simulink model "px42LoopCtrQGCGPS202203131707"  (R2022a)
settings: Solver=FixedStepDiscrete  StartTime=0.0  StopTime=inf  FixedStep=0.005  RelTol=1e-3  EnableMultiTasking=on
InitFcn:
  | I_x = 0.00478;
  | I_y = 0.00502;
  | I_z = 0.00736;
  | m=1;
  | L=0.11667;
undefined symbols (not defined in the file): alt, cog_rad, dev, DiscIntNeverNeededParam, eph, epv, fix_type, lat, lon, m_to_mm, Main, ms_to_cms, pwm_output0, ref_height, ref_lat, ref_lon, SampleTime, satellites_used, time_utc_usec, vel_d_m_s, vel_e_m_s, vel_m_s, vel_n_m_s, vx, vy, vz, x, y, z
libraries: simulink x26, px4uORBlib x5, sensorgpslib x1, px4lib x1, slpidlib x1, sharedtransform x1, px4Sensorslib x1
(part 3 of 3)

== system px42LoopCtrQGCGPS202203131707/Attitude controller/Subsystem1/Subsystem1/Subsystem ==
  Add1 : Sum
  Data Store Read : DataStoreRead  DataStoreName=t  IndexOptions=Index vector (dialog)  Indices=1  OutputSizes=1
  Fcn : Fcn  Expr=u(1)/(u(2)-u(3))
  Mux1 : Mux  Inputs=3
  Scope : Scope
  Switch : Switch  Threshold=5  SaturateOnIntegerOverflow=off  InputSameDT=off
  T : Constant  Value=5
  ch : Constant  Value=3
  r : Constant
  t : Constant  Value=0
  H : Outport
  wires:
  r/1 -> Add1/1
  Data Store Read/1 -> Switch/2, Mux1/3
  Mux1/1 -> Fcn/1
  ch/1 -> Mux1/1
  t/1 -> Switch/1
  T/1 -> Mux1/2
  Add1/1 -> H/1
  Fcn/1 -> Switch/3
  Switch/1 -> Scope/1, Add1/2

== system px42LoopCtrQGCGPS202203131707/Attitude controller/Subsystem6/Subsystem1/Subsystem ==
  Abs : Abs  SaturateOnIntegerOverflow=off
  Add : Sum  Inputs=+-
  Add1 : Sum
  Compare To Constant1 : simulink/Logic and Bit Operations/Compare To Constant  relop=>=  const=pi/36  OutDataTypeStr=boolean
  Data Store Memory : DataStoreMemory  DataStoreName=start_time_roll  ReadBeforeWriteMsg=warning  WriteAfterWriteMsg=warning  WriteAfterReadMsg=warning  ShowAdditionalParam=off
  Data Store Read : DataStoreRead  DataStoreName=t  IndexOptions=Index vector (dialog)  Indices=1  OutputSizes=1
  Data Store Read1 : DataStoreRead  DataStoreName=e_pitch_roll  IndexOptions=Index vector (dialog)  Indices=1  OutputSizes=1
  Data Store Read3 : DataStoreRead  DataStoreName=start_time_roll  IndexOptions=Index vector (dialog)  Indices=1  OutputSizes=1
  Data Store Read4 : DataStoreRead  DataStoreName=start_time_roll  IndexOptions=Index vector (dialog)  Indices=1  OutputSizes=1
  Display : Display
  Fcn : Fcn  Expr=u(1)/(u(2)-u(3))
  MATLAB Function : MATLAB Function  TreatAsAtomicUnit=on
  Mux1 : Mux  Inputs=3
  Scope : Scope
  T : Constant  Value=5
  ch : Constant  Value=2
  r : Constant  Value=6.001388888888889
  start_time : Subsystem
  t : Constant  Value=0
  H : Outport
  wires:
  MATLAB Function/1(y) -> Scope/1, Add1/2
  Compare To Constant1/1 -> MATLAB Function/1(e)
  Fcn/1 -> MATLAB Function/4(y1)
  t/1 -> MATLAB Function/5(y2)
  Data Store Read4/1 -> Display/1
  Data Store Read3/1 -> Add/2, MATLAB Function/3(s_t)
  Mux1/1 -> Fcn/1
  Add/1 -> Mux1/3
  ch/1 -> Mux1/1
  Data Store Read/1 -> Add/1, MATLAB Function/2(t)
  T/1 -> Mux1/2
  Abs/1 -> Compare To Constant1/1
  Data Store Read1/1 -> Abs/1
  Add1/1 -> H/1
  r/1 -> Add1/1

== system px42LoopCtrQGCGPS202203131707/Attitude controller/Subsystem7/Subsystem1/Subsystem ==
  Abs : Abs  SaturateOnIntegerOverflow=off
  Add : Sum  Inputs=+-
  Add1 : Sum
  Compare To Constant1 : simulink/Logic and Bit Operations/Compare To Constant  relop=>=  const=pi/36  OutDataTypeStr=boolean
  Data Store Memory : DataStoreMemory  DataStoreName=start_time_yaw  ReadBeforeWriteMsg=warning  WriteAfterWriteMsg=warning  WriteAfterReadMsg=warning  ShowAdditionalParam=off
  Data Store Read : DataStoreRead  DataStoreName=t  IndexOptions=Index vector (dialog)  Indices=1  OutputSizes=1
  Data Store Read1 : DataStoreRead  DataStoreName=e_pitch_yaw  IndexOptions=Index vector (dialog)  Indices=1  OutputSizes=1
  Data Store Read3 : DataStoreRead  DataStoreName=start_time_yaw  IndexOptions=Index vector (dialog)  Indices=1  OutputSizes=1
  Data Store Read4 : DataStoreRead  DataStoreName=start_time_yaw  IndexOptions=Index vector (dialog)  Indices=1  OutputSizes=1
  Display : Display
  Fcn : Fcn  Expr=u(1)/(u(2)-u(3))
  MATLAB Function : MATLAB Function  TreatAsAtomicUnit=on
  Mux1 : Mux  Inputs=3
  Scope : Scope
  T : Constant  Value=5
  ch : Constant  Value=2
  r : Constant  Value=8.00109649122807
  start_time : Subsystem
  t : Constant  Value=0
  H : Outport
  wires:
  MATLAB Function/1(y) -> Scope/1, Add1/2
  Compare To Constant1/1 -> MATLAB Function/1(e)
  Fcn/1 -> MATLAB Function/4(y1)
  t/1 -> MATLAB Function/5(y2)
  Data Store Read4/1 -> Display/1
  Data Store Read3/1 -> Add/2, MATLAB Function/3(s_t)
  Mux1/1 -> Fcn/1
  Add/1 -> Mux1/3
  ch/1 -> Mux1/1
  Data Store Read/1 -> Add/1, MATLAB Function/2(t)
  T/1 -> Mux1/2
  Abs/1 -> Compare To Constant1/1
  Data Store Read1/1 -> Abs/1
  Add1/1 -> H/1
  r/1 -> Add1/1

== system px42LoopCtrQGCGPS202203131707/Attitude controller/Subsystem/Subsystem1/Subsystem/start_time ==
  Abs1 : Abs  SaturateOnIntegerOverflow=off
  Abs2 : Abs  Commented=on  SaturateOnIntegerOverflow=off
  Add : Sum  Inputs=+-
  Add2 : Sum  Commented=on  Inputs=+-
  Compare To Constant1 : simulink/Logic and Bit Operations/Compare To Constant  relop=>=  const=4.6  OutDataTypeStr=boolean
  Compare To Constant2 : simulink/Logic and Bit Operations/Compare To Constant  relop=>=  const=pi/36  OutDataTypeStr=boolean
  Compare To Constant4 : simulink/Logic and Bit Operations/Compare To Constant  Commented=on  relop=>=  const=pi/36  OutDataTypeStr=boolean
  Compare To Constant5 : simulink/Logic and Bit Operations/Compare To Constant  Commented=on  relop=>=  const=5  OutDataTypeStr=boolean
  Data Store Read : DataStoreRead  DataStoreName=t  IndexOptions=Index vector (dialog)  Indices=1  OutputSizes=1
  Data Store Read2 : DataStoreRead  DataStoreName=e_pitch  IndexOptions=Index vector (dialog)  Indices=1  OutputSizes=1
  Data Store Read3 : DataStoreRead  DataStoreName=start_time  IndexOptions=Index vector (dialog)  Indices=1  OutputSizes=1
  Data Store Read5 : DataStoreRead  Commented=on  DataStoreName=e_pitch  IndexOptions=Index vector (dialog)  Indices=1  OutputSizes=1
  Data Store Read6 : DataStoreRead  Commented=on  DataStoreName=t  IndexOptions=Index vector (dialog)  Indices=1  OutputSizes=1
  Data Store Read7 : DataStoreRead  Commented=on  DataStoreName=start_time  IndexOptions=Index vector (dialog)  Indices=1  OutputSizes=1
  Logical Operator : Logic  AllPortsSameDT=off  OutDataTypeStr=boolean
  Logical Operator1 : Logic  Commented=on  AllPortsSameDT=off  OutDataTypeStr=boolean
  Subsystem : Subsystem
  Subsystem1 : Subsystem  Commented=on
  wires:
  Data Store Read7/1 -> Add2/2
  Abs1/1 -> Compare To Constant2/1
  Data Store Read2/1 -> Abs1/1
  Logical Operator1/1 -> Subsystem1/Trigger
  Compare To Constant5/1 -> Logical Operator1/2
  Add2/1 -> Compare To Constant5/1
  Compare To Constant4/1 -> Logical Operator1/1
  Data Store Read5/1 -> Abs2/1
  Data Store Read6/1 -> Add2/1
  Abs2/1 -> Compare To Constant4/1
  Data Store Read3/1 -> Add/2
  Data Store Read/1 -> Add/1
  Add/1 -> Compare To Constant1/1
  Compare To Constant2/1 -> Logical Operator/1
  Compare To Constant1/1 -> Logical Operator/2
  Logical Operator/1 -> Subsystem/Trigger

== system px42LoopCtrQGCGPS202203131707/Attitude controller/Subsystem6/Subsystem1/Subsystem/start_time ==
  Abs1 : Abs  SaturateOnIntegerOverflow=off
  Abs2 : Abs  Commented=on  SaturateOnIntegerOverflow=off
  Add : Sum  Inputs=+-
  Add2 : Sum  Commented=on  Inputs=+-
  Compare To Constant1 : simulink/Logic and Bit Operations/Compare To Constant  relop=>=  const=4.6  OutDataTypeStr=boolean
  Compare To Constant2 : simulink/Logic and Bit Operations/Compare To Constant  relop=>=  const=pi/36  OutDataTypeStr=boolean
  Compare To Constant4 : simulink/Logic and Bit Operations/Compare To Constant  Commented=on  relop=>=  const=pi/36  OutDataTypeStr=boolean
  Compare To Constant5 : simulink/Logic and Bit Operations/Compare To Constant  Commented=on  relop=>=  const=5  OutDataTypeStr=boolean
  Data Store Read : DataStoreRead  DataStoreName=t  IndexOptions=Index vector (dialog)  Indices=1  OutputSizes=1
  Data Store Read2 : DataStoreRead  DataStoreName=e_pitch_roll  IndexOptions=Index vector (dialog)  Indices=1  OutputSizes=1
  Data Store Read3 : DataStoreRead  DataStoreName=start_time_roll  IndexOptions=Index vector (dialog)  Indices=1  OutputSizes=1
  Data Store Read5 : DataStoreRead  Commented=on  DataStoreName=e_pitch  IndexOptions=Index vector (dialog)  Indices=1  OutputSizes=1
  Data Store Read6 : DataStoreRead  Commented=on  DataStoreName=t  IndexOptions=Index vector (dialog)  Indices=1  OutputSizes=1
  Data Store Read7 : DataStoreRead  Commented=on  DataStoreName=start_time  IndexOptions=Index vector (dialog)  Indices=1  OutputSizes=1
  Logical Operator : Logic  AllPortsSameDT=off  OutDataTypeStr=boolean
  Logical Operator1 : Logic  Commented=on  AllPortsSameDT=off  OutDataTypeStr=boolean
  Subsystem : Subsystem
  Subsystem1 : Subsystem  Commented=on
  wires:
  Logical Operator/1 -> Subsystem/Trigger
  Compare To Constant1/1 -> Logical Operator/2
  Compare To Constant2/1 -> Logical Operator/1
  Add/1 -> Compare To Constant1/1
  Data Store Read/1 -> Add/1
  Data Store Read3/1 -> Add/2
  Abs2/1 -> Compare To Constant4/1
  Data Store Read6/1 -> Add2/1
  Data Store Read5/1 -> Abs2/1
  Compare To Constant4/1 -> Logical Operator1/1
  Add2/1 -> Compare To Constant5/1
  Compare To Constant5/1 -> Logical Operator1/2
  Logical Operator1/1 -> Subsystem1/Trigger
  Data Store Read2/1 -> Abs1/1
  Abs1/1 -> Compare To Constant2/1
  Data Store Read7/1 -> Add2/2

== system px42LoopCtrQGCGPS202203131707/Attitude controller/Subsystem7/Subsystem1/Subsystem/start_time ==
  Abs1 : Abs  SaturateOnIntegerOverflow=off
  Abs2 : Abs  Commented=on  SaturateOnIntegerOverflow=off
  Add : Sum  Inputs=+-
  Add2 : Sum  Commented=on  Inputs=+-
  Compare To Constant1 : simulink/Logic and Bit Operations/Compare To Constant  relop=>=  const=4.8  OutDataTypeStr=boolean
  Compare To Constant2 : simulink/Logic and Bit Operations/Compare To Constant  relop=>=  const=pi/36  OutDataTypeStr=boolean
  Compare To Constant4 : simulink/Logic and Bit Operations/Compare To Constant  Commented=on  relop=>=  const=pi/36  OutDataTypeStr=boolean
  Compare To Constant5 : simulink/Logic and Bit Operations/Compare To Constant  Commented=on  relop=>=  const=5  OutDataTypeStr=boolean
  Data Store Read : DataStoreRead  DataStoreName=t  IndexOptions=Index vector (dialog)  Indices=1  OutputSizes=1
  Data Store Read2 : DataStoreRead  DataStoreName=e_pitch_yaw  IndexOptions=Index vector (dialog)  Indices=1  OutputSizes=1
  Data Store Read3 : DataStoreRead  DataStoreName=start_time_yaw  IndexOptions=Index vector (dialog)  Indices=1  OutputSizes=1
  Data Store Read5 : DataStoreRead  Commented=on  DataStoreName=e_pitch  IndexOptions=Index vector (dialog)  Indices=1  OutputSizes=1
  Data Store Read6 : DataStoreRead  Commented=on  DataStoreName=t  IndexOptions=Index vector (dialog)  Indices=1  OutputSizes=1
  Data Store Read7 : DataStoreRead  Commented=on  DataStoreName=start_time  IndexOptions=Index vector (dialog)  Indices=1  OutputSizes=1
  Logical Operator : Logic  AllPortsSameDT=off  OutDataTypeStr=boolean
  Logical Operator1 : Logic  Commented=on  AllPortsSameDT=off  OutDataTypeStr=boolean
  Subsystem : Subsystem
  Subsystem1 : Subsystem  Commented=on
  wires:
  Logical Operator/1 -> Subsystem/Trigger
  Compare To Constant1/1 -> Logical Operator/2
  Compare To Constant2/1 -> Logical Operator/1
  Add/1 -> Compare To Constant1/1
  Data Store Read/1 -> Add/1
  Data Store Read3/1 -> Add/2
  Abs2/1 -> Compare To Constant4/1
  Data Store Read6/1 -> Add2/1
  Data Store Read5/1 -> Abs2/1
  Compare To Constant4/1 -> Logical Operator1/1
  Add2/1 -> Compare To Constant5/1
  Compare To Constant5/1 -> Logical Operator1/2
  Logical Operator1/1 -> Subsystem1/Trigger
  Data Store Read2/1 -> Abs1/1
  Abs1/1 -> Compare To Constant2/1
  Data Store Read7/1 -> Add2/2

== system px42LoopCtrQGCGPS202203131707/Attitude controller/Subsystem/Subsystem1/Subsystem/start_time/Subsystem ==
  Trigger : TriggerPort  VariantControl=Variant  PortDimensions=1
  Data Store Read2 : DataStoreRead  DataStoreName=t  IndexOptions=Index vector (dialog)  Indices=1  OutputSizes=1
  Data Store Write : DataStoreWrite  DataStoreName=start_time  IndexOptions=Index vector (dialog)  Indices=1  OutputSizes=1
  wires:
  Data Store Read2/1 -> Data Store Write/1

== system px42LoopCtrQGCGPS202203131707/Attitude controller/Subsystem/Subsystem1/Subsystem/start_time/Subsystem1 ==
  Trigger : TriggerPort  VariantControl=Variant  PortDimensions=1
  Data Store Read2 : DataStoreRead  DataStoreName=t  IndexOptions=Index vector (dialog)  Indices=1  OutputSizes=1
  Data Store Write : DataStoreWrite  DataStoreName=start_time  IndexOptions=Index vector (dialog)  Indices=1  OutputSizes=1
  wires:
  Data Store Read2/1 -> Data Store Write/1

== system px42LoopCtrQGCGPS202203131707/Attitude controller/Subsystem6/Subsystem1/Subsystem/start_time/Subsystem ==
  Trigger : TriggerPort  VariantControl=Variant  PortDimensions=1
  Data Store Read2 : DataStoreRead  DataStoreName=t  IndexOptions=Index vector (dialog)  Indices=1  OutputSizes=1
  Data Store Write : DataStoreWrite  DataStoreName=start_time_roll  IndexOptions=Index vector (dialog)  Indices=1  OutputSizes=1
  wires:
  Data Store Read2/1 -> Data Store Write/1

== system px42LoopCtrQGCGPS202203131707/Attitude controller/Subsystem6/Subsystem1/Subsystem/start_time/Subsystem1 ==
  Trigger : TriggerPort  VariantControl=Variant  PortDimensions=1
  Data Store Read2 : DataStoreRead  DataStoreName=t  IndexOptions=Index vector (dialog)  Indices=1  OutputSizes=1
  Data Store Write : DataStoreWrite  DataStoreName=start_time  IndexOptions=Index vector (dialog)  Indices=1  OutputSizes=1
  wires:
  Data Store Read2/1 -> Data Store Write/1

== system px42LoopCtrQGCGPS202203131707/Attitude controller/Subsystem7/Subsystem1/Subsystem/start_time/Subsystem ==
  Trigger : TriggerPort  VariantControl=Variant  PortDimensions=1
  Data Store Read2 : DataStoreRead  DataStoreName=t  IndexOptions=Index vector (dialog)  Indices=1  OutputSizes=1
  Data Store Write : DataStoreWrite  DataStoreName=start_time_yaw  IndexOptions=Index vector (dialog)  Indices=1  OutputSizes=1
  wires:
  Data Store Read2/1 -> Data Store Write/1

== system px42LoopCtrQGCGPS202203131707/Attitude controller/Subsystem7/Subsystem1/Subsystem/start_time/Subsystem1 ==
  Trigger : TriggerPort  VariantControl=Variant  PortDimensions=1
  Data Store Read2 : DataStoreRead  DataStoreName=t  IndexOptions=Index vector (dialog)  Indices=1  OutputSizes=1
  Data Store Write : DataStoreWrite  DataStoreName=start_time  IndexOptions=Index vector (dialog)  Indices=1  OutputSizes=1
  wires:
  Data Store Read2/1 -> Data Store Write/1

== matlab function px42LoopCtrQGCGPS202203131707/MATLAB Function2 ==
  data: q_x input; u output; q_y input; q_z input
function u = fcn(q_x,q_y,q_z)
m = 1;
g = 9.8;
u=(sqrt((q_x^2)+(q_y^2)+(q_z+g)^2))*m;

== matlab function px42LoopCtrQGCGPS202203131707/MATLAB Function3 ==
  data: qx input; qy input; qz input; psi_d input; u input; phi_d output; theta_d output
function [phi_d,theta_d] = fcn(qx,qy,qz,psi_d,u)
g = 9.8;
m =1;

a = asin(m*(qx*sin(psi_d)-qy*cos(psi_d))/u);
b = atan((qx*cos(psi_d)+qy*sin(psi_d))/(g+qz));
if a>pi/18
    a = pi/18;
elseif a<-pi/18
    a = -pi/18;   
end
if b>pi/18
    b = pi/18;
elseif b<-pi/18
    b = -pi/18;
end
phi_d = a;
theta_d = b;
% p_d = a/100;
% t_d = b/100;

== matlab function px42LoopCtrQGCGPS202203131707/MATLAB Function1 ==
  data: phi input; theta input; psi input; dd_x output; dd_y output; u input; dd_z output
function [dd_x,dd_y,dd_z] = fcn(phi,theta,psi,u)
m = 1;
g = 9.8;
dd_x = -u*(cos(phi)*sin(theta)*cos(psi)+sin(phi)*sin(psi))/m;
dd_y = -u*(cos(phi)*sin(theta)*sin(psi)-sin(phi)*cos(psi))/m;
dd_z = -u*cos(theta)*cos(phi)/m+g;

== matlab function px42LoopCtrQGCGPS202203131707/MATLAB Function4 ==
  data: q_x input; u output; q_y input; q_z input
function u = fcn(q_x,q_y,q_z)
m = 1;
g = 9.8;
u =m(q_x^2+q_y^2+(q_z+g)^2)^(1/2);

== matlab function px42LoopCtrQGCGPS202203131707/Attitude controller/Subsystem2/MATLAB Function ==
  data: u input; y output
function y = fcn(u)

y = erf(u);

== matlab function px42LoopCtrQGCGPS202203131707/Attitude controller/Subsystem3/MATLAB Function ==
  data: u input; y output
function y = fcn(u)

y = erf(u);

== matlab function px42LoopCtrQGCGPS202203131707/Attitude controller/Subsystem/Subsystem1/Subsystem/MATLAB Function ==
  data: e input; y output; t input; s_t input; y1 input; y2 input
function y = fcn(e,t,s_t,y1,y2)
if t<4.6
    y=y2;
elseif e>0&&t-s_t<=4.6&&t>4.6
    y=y1;
elseif e>0&&t-s_t>4.6
    y=y2;
elseif e<=0&&t-s_t<=4.6&&t>4.6
    y=y1;
elseif e<=0&&t-s_t>4.6
    y=y2;
else
    y=y2;
end

== matlab function px42LoopCtrQGCGPS202203131707/Attitude controller/Subsystem6/Subsystem1/Subsystem/MATLAB Function ==
  data: e input; y output; t input; s_t input; y1 input; y2 input
function y = fcn(e,t,s_t,y1,y2)
if t<4.6
    y=y2;
elseif e>0&&t-s_t<=4.6&&t>4.6
    y=y1;
elseif e>0&&t-s_t>4.6
    y=y2;
elseif e<=0&&t-s_t<=4.6&&t>4.6
    y=y1;
elseif e<=0&&t-s_t>4.6
    y=y2;
else
    y=y2;
end

== matlab function px42LoopCtrQGCGPS202203131707/Attitude controller/Subsystem7/Subsystem1/Subsystem/MATLAB Function ==
  data: e input; y output; t input; s_t input; y1 input; y2 input
function y = fcn(e,t,s_t,y1,y2)
if t<4.6
    y=y2;
elseif e>0&&t-s_t<=4.6&&t>4.6
    y=y1;
elseif e>0&&t-s_t>4.6
    y=y2;
elseif e<=0&&t-s_t<=4.6&&t>4.6
    y=y1;
elseif e<=0&&t-s_t>4.6
    y=y2;
else
    y=y2;
end
